simulink model "rep3_transc_analysis_response"  (R2015a)
settings: Solver=ode4  StartTime=0.0  StopTime=100  FixedStep=0.1  RelTol=1e-3
values from neighbouring files (symbols this model uses):
  c1 = 1.6    [rep3_transc_analysis_init.m]
  c2 = 0.12    [rep3_transc_analysis_init.m]
  c3 = 2.6    [rep3_transc_analysis_init.m]
  c4 = 0.06    [rep3_transc_analysis_init.m]
  K_D = 1    [rep3_transc_analysis_init.m]
  mRNA_init = 0.5    [rep3_transc_analysis_init.m]
  n0 = 0.5    [rep3_transc_analysis_init.m]
  n1 = 2    [rep3_transc_analysis_init.m]
  n2 = 4    [rep3_transc_analysis_init.m]
libraries: fuzblock x3, simulink x1
settings Model: Creator=Jure Bordon  LastModifiedBy=jureb
settings DataIOCC: InspectSignalLogs=on
settings DebuggingCC: UnderspecifiedInitializationDetection=Classic  MergeDetectMultiDrivingBlocksExec=none  SolverPrmCheckMsg=warning  StateNameClashWarn=warning

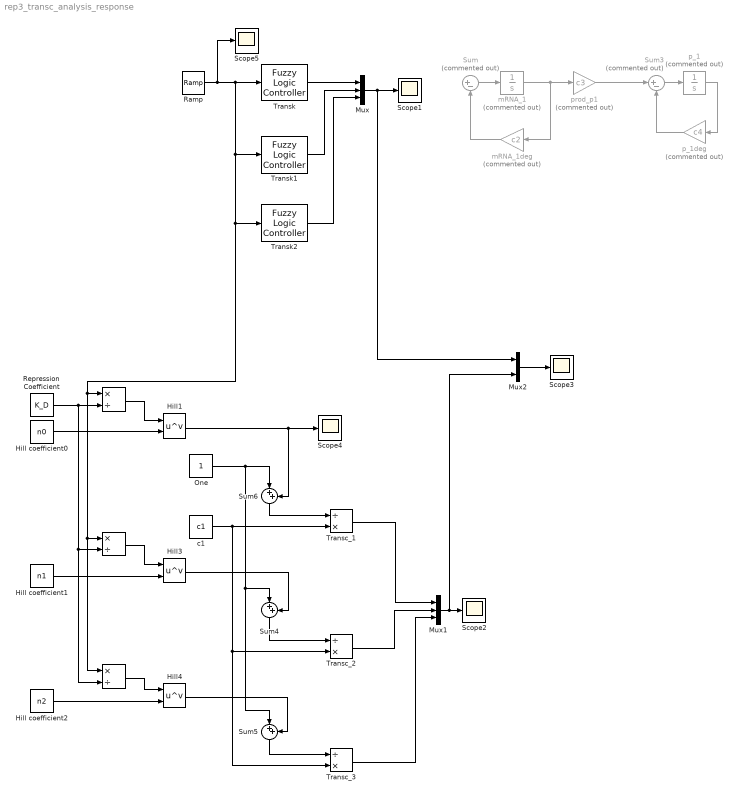
== system rep3_transc_analysis_response ==
  " " : Product  Inputs=*/
  " " : Product  Inputs=*/
  " " : Product  Inputs=*/
  Hill coefficient0 : Constant  Value=n0
  Hill coefficient1 : Constant  Value=n1
  Hill coefficient2 : Constant  Value=n2
  Hill1 : Math  Operator=pow  SaturateOnIntegerOverflow=on
  Hill3 : Math  Operator=pow  SaturateOnIntegerOverflow=on
  Hill4 : Math  Operator=pow  SaturateOnIntegerOverflow=on
  Mux : Mux  Inputs=3
  Mux1 : Mux  Inputs=3
  Mux2 : Mux  Inputs=2
  One : Constant
  Ramp : simulink/Sources/Ramp  slope=4  start=0  X0=0
  Repression Coefficient : Constant  Value=K_D
  Scope{1..5} (5 alike) : Scope
      Scope1 settings: TimeRange=100  YMin=0  YMax=1.5  SaveName=mRNA_FL
      Scope2 settings: TimeRange=100  YMin=0  YMax=1.5  SaveName=mRNA_ODE
      Scope3 settings: TimeRange=100  YMin=0  YMax=1.5  SaveName=mRNAChange2
      Scope4 settings: TimeRange=100  YMin=0  YMax=1.5  SaveName=mRNAChange3
      Scope5 settings: TimeRange=100  YMin=0  YMax=1.5  SaveName=mRNAChange4
  Sum : Sum  Commented=on  Inputs=|+-
  Sum3 : Sum  Commented=on  Inputs=|+-
  Sum4 : Sum  Inputs=|++
  Sum5 : Sum  Inputs=|++
  Sum6 : Sum  Inputs=|++
  Transc_1 : Product  Inputs=/*
  Transc_2 : Product  Inputs=/*
  Transc_3 : Product  Inputs=/*
  Transk : fuzblock/Fuzzy Logic  Controller  fis=Transk0
  Transk1 : fuzblock/Fuzzy Logic  Controller  fis=Transk1
  Transk2 : fuzblock/Fuzzy Logic  Controller  fis=Transk2
  c1 : Constant  Value=c1
  mRNA_1 : Integrator  Commented=on  InitialCondition=mRNA_init + 0.5  LimitOutput=on  LowerSaturationLimit=0
  mRNA_1deg : Gain  Commented=on  Gain=c2
  p_1 : Integrator  Commented=on  LimitOutput=on  LowerSaturationLimit=0
  p_1deg : Gain  Commented=on  Gain=c4
  prod_p1 : Gain  Commented=on  Gain=c3
  wires:
  Sum/1 -> mRNA_1/1
  Sum3/1 -> p_1/1
  p_1/1 -> p_1deg/1
  p_1deg/1 -> Sum3/2
  mRNA_1/1 -> prod_p1/1, mRNA_1deg/1
  mRNA_1deg/1 -> Sum/2
  prod_p1/1 -> Sum3/1
  Mux/1 -> Mux2/1, Scope1/1
  Transk/1 -> Mux/1
  Transk1/1 -> Mux/2
  Transk2/1 -> Mux/3
  One/1 -> Sum4/1, Sum5/1, Sum6/1
  Hill1/1 -> Scope4/1, Sum6/2
  Sum6/1 -> Transc_1/1
  c1/1 -> Transc_3/2, Transc_2/2, Transc_1/2
  Sum4/1 -> Transc_2/1
  Hill3/1 -> Sum4/2
  Hill coefficient2/1 -> Hill4/2
  Hill4/1 -> Sum5/2
  Sum5/1 -> Transc_3/1
  Mux1/1 -> Mux2/2, Scope2/1
  Transc_1/1 -> Mux1/1
  Transc_2/1 -> Mux1/2
  Transc_3/1 -> Mux1/3
  Mux2/1 -> Scope3/1
  Hill coefficient0/1 -> Hill1/2
  Ramp/1 -> Scope5/1, Transk/1, Transk1/1, Transk2/1, " "/1, " "/1, " "/1
  Hill coefficient1/1 -> Hill3/2
  " "/1 -> Hill1/1
  Repression Coefficient/1 -> " "/2, " "/2, " "/2
  " "/1 -> Hill3/1
  " "/1 -> Hill4/1
